simulink model "Single_Phase_Fully_Controlled_Bridge_Rectifier"  (Simulink 7.5)
settings: Solver=ode45  StartTime=0.0  StopTime=3  RelTol=1e-3
libraries: powerlib x11
settings Model: Creator=lm  LastModifiedBy=lm

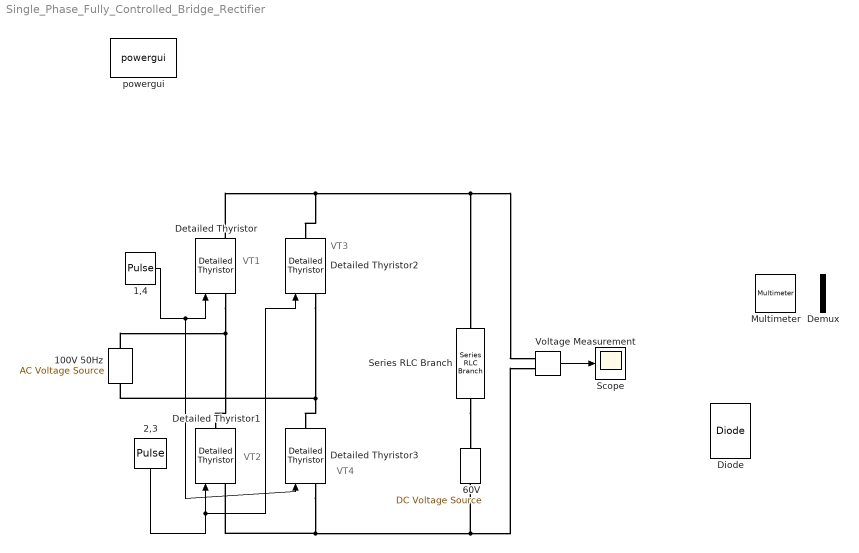
== system Single_Phase_Fully_Controlled_Bridge_Rectifier ==
  note: VT1
  note: VT3
  note: VT2
  note: VT4
  1,4 : DiscretePulseGenerator  PulseType=Time based  Amplitude=10  Period=0.02  PulseWidth=5  PhaseDelay=(2/12)*0.02  SampleTime=1
  100V 50Hz : powerlib/Electrical Sources/AC Voltage Source  DialogController=POWERSYS.PowerSysDialog  SystemSampleTime=-1  Amplitude=100*sqrt(2)  Phase=0  Frequency=50  SampleTime=0  Measurements=Voltage
  2,3 : DiscretePulseGenerator  PulseType=Time based  Amplitude=10  Period=0.02  PulseWidth=5  PhaseDelay=(2/12)*0.02+0.01  SampleTime=1
  60V : powerlib/Electrical Sources/DC Voltage Source  DialogController=POWERSYS.PowerSysDialog  SystemSampleTime=-1  Amplitude=60  Measurements=None
  Demux : Demux  Outputs=3
  Detailed Thyristor : powerlib/Power Electronics/Detailed Thyristor  DialogController=POWERSYS.PowerSysDialog  SystemSampleTime=-1  Ron=0.001  Lon=1e-3  Vf=0.8  IL=0.1  Tq=100e-6  IC=0  Rs=500  Cs=250e-9  Measurements=on
  Detailed Thyristor1 : powerlib/Power Electronics/Detailed Thyristor  DialogController=POWERSYS.PowerSysDialog  SystemSampleTime=-1  Ron=0.001  Lon=1e-3  Vf=0.8  IL=0.1  Tq=100e-6  IC=0  Rs=500  Cs=250e-9  Measurements=off
  Detailed Thyristor2 : powerlib/Power Electronics/Detailed Thyristor  DialogController=POWERSYS.PowerSysDialog  SystemSampleTime=-1  Ron=0.001  Lon=1e-3  Vf=0.8  IL=0.1  Tq=100e-6  IC=0  Rs=500  Cs=250e-9  Measurements=off
  Detailed Thyristor3 : powerlib/Power Electronics/Detailed Thyristor  DialogController=POWERSYS.PowerSysDialog  SystemSampleTime=-1  Ron=0.001  Lon=1e-3  Vf=0.8  IL=0.1  Tq=100e-6  IC=0  Rs=500  Cs=250e-9  Measurements=off
  Diode : powerlib/Power Electronics/Diode  DialogController=POWERSYS.PowerSysDialog  SystemSampleTime=-1  Ron=0.001  Lon=0  Vf=0.8  IC=0  UseSnubber=off  Rs=500  Cs=250e-9  Measurements=on
  Multimeter : powerlib/Measurements/Multimeter  SystemSampleTime=-1  PhasorSimulation=off  OutputType=Complex  sel=[2 1 3]  L=3  Gain=[1 1 1]  yselected={'Usrc: 100V 50Hz','Ub: Series RLC Branch','Ib: Series RLC Branch'};  PSBOutputType=1  PSBequivalent=0  AxesSetting=[0,0.1,-100,100]  Display=0  SavedBlockNames=-11
  Scope : Scope
      settings: TimeRange=0.06581979125379842  YMin=0  YMax=150
  Series RLC Branch : powerlib/Elements/Series RLC Branch  DialogController=POWERSYS.PowerSysDialog  PhysicalDomain=powersysdomain  SubClassName=unknown  LeftPortType=p1  RightPortType=p1  LConnTagsString=__new0  RConnTagsString=__new0  BranchType=R  Resistance=5  Inductance=1  SetiL0=off  InitialCurrent=0  Capacitance=1e-6  Setx0=off  InitialVoltage=0  Measurements=Branch voltage and current
  Voltage Measurement : powerlib/Measurements/Voltage Measurement  DialogController=POWERSYS.PowerSysDialog  SystemSampleTime=-1  PhasorSimulation=off  OutputType=Complex  PSBequivalent=0
  powergui : powerlib/powergui  Priority=1  SystemSampleTime=-1  SimulationMode=Discrete  SampleTime=50e-6  frequency=60  SPID=off  DisableSnubberDevices=off  DisableRonSwitches=off  DisableVfSwitches=off  SwTol=0  Interpol=off  frequencyindice=50  echomessages=off  HookPort=off  DisplayEquations=off  FunctionMessages=off  EnableUseOfTLC=off  x0status=blocks  RestoreLinks=warning  ResistiveCurrentMeasurement=off  Ylog=off  Xlog=on  ShowGrid=off  save=off  variable=ZData  ZoomFFT=off  StartTime=0.0  cycles=1  DisplayStyle=1  FreqAxis=off  MaxFrequency=1000  frequencyindicesteady=1  display=off  methode=off
  wires:
  1,4/1 -> Detailed Thyristor/1, Detailed Thyristor3/1
  2,3/1 -> Detailed Thyristor1/1, Detailed Thyristor2/1
  Voltage Measurement/1 -> Scope/1
  connections:
  Detailed Thyristor/LConn1 -- Detailed Thyristor1/RConn1 -- 100V 50Hz/RConn1
  Detailed Thyristor3/LConn1 -- Detailed Thyristor1/LConn1 -- 60V/LConn1 -- Voltage Measurement/LConn2
  Detailed Thyristor/RConn1 -- Detailed Thyristor2/RConn1 -- Series RLC Branch/LConn1 -- Voltage Measurement/LConn1
  Detailed Thyristor2/LConn1 -- Detailed Thyristor3/RConn1 -- 100V 50Hz/LConn1
  Series RLC Branch/RConn1 -- 60V/RConn1
